simulink model "BMSStateMachine"  (R2023b)
settings: Solver=FixedStepDiscrete  StartTime=0.0  StopTime=10000  RelTol=1e-3
model workspace (MAT data in the model file):
  CV_Gain = 0.20000000298
  HighTempLimit = 50
  I_cc = 30
  LowTempLimit = 5
  MaxCellVoltThrsld = 4.19999980927
  OverCellVoltageLimit = 4.19999980927
  SnsrFltThld = 0.252
  UnderCellVoltageLimit = 2.5
  contactorTime = 200
  currentFactor = 10
  noCurrent = 0
  timeoutContactor = 1
  timeoutCurrent = 1
  vRatio = 0.949999988079
  voltThreshold = 4.09999990463
settings Model: DataDictionary=VirtualVehicleTemplate.sldd  ModifiedByFormat=The MathWorks, Inc.  ExtModeTrigDuration=5  Creator=The MathWorks, Inc.  LastModifiedBy=The MathWorks, Inc.
settings SolverCC: AlgebraicLoopSolver=TrustRegion  PositivePriorityOrder=on  AutoInsertRateTranBlk=on  MaxZcPerStep=1
settings DataIOCC: ExternalInput=Battery  SaveOutput=off  SaveTime=off  SignalLoggingName=logsOut
settings OptimizationCC: BlockReduction=off  DefaultParameterBehavior=Inlined  UseFloatMulNetSlope=on  DefaultUnderspecifiedDataType=single  OptimizeBlockIOStorage=off  EnhancedBackFolding=on  PassReuseOutputArgsThreshold=0  ZeroExternalMemoryAtStartup=off  ZeroInternalMemoryAtStartup=off  EfficientFloat2IntCast=on  MaxStackSize=64  OptimizeBlockOrder=speed  DifferentSizesBufferReuse=on
settings DebuggingCC: SignalInfNanChecking=error  SaveWithParameterizedLinksMsg=none  CheckExecutionContextPreStartOutputMsg=on  IntegerOverflowMsg=error  ParameterPrecisionLossMsg=none  ParameterTunabilityLossMsg=error  UnconnectedInputMsg=warning  UnconnectedOutputMsg=warning  UnconnectedLineMsg=warning  AssertControl=DisableAll  PregeneratedLibrarySubsystemCodeDiagnostic=none  SubsystemReferenceDiagnosticForUnitTest=warning  SFUnexpectedBacktrackingDiag=warning  SFNoUnconditionalDefaultTransitionDiag=warning  SFExecutionAtInitializationDiag=none  ArithmeticOperatorsInVariantConditions=warning
settings HardwareCC: ProdBitPerLong=64  ProdLongLongMode=on  ProdHWDeviceType=Intel->x86-64 (Linux 64)
settings ModelReferenceCC: EnableRefExpFcnMdlSchedulingChecks=on  ModelReferenceNumInstancesAllowed=Single  PropagateSignalLabelsOutOfModel=off
settings SFSimCC: SimUseLocalCustomCode=off  MATLABDynamicMemAlloc=off  CustomCodeUndefinedFunction=UseInterfaceOnly
settings RTWCC: GenerateReport=on  RTWUseLocalCustomCode=off  Toolchain=Simulink Real-Time Toolchain  BuildConfiguration=Faster Runs  TargetLang=C++  DLArmComputeVersion=19.05
settings CodeAppCC: ForceParamTrailComments=on  MaxIdLength=51  OperatorAnnotations=on  MangleLength=4
settings GRTTargetCC: TargetLangStandard=C++03 (ISO)  CodeInterfacePackaging=C++ class
settings ConfigComp: CovMetricSettings=dcw  CovSaveCumulativeToWorkspaceVar=on  CovSaveSingleToWorkspaceVar=on  CovExternalEMLEnable=off  CovSFcnEnable=off  DVMode=DesignErrorDetection  DVMaxProcessTime=7000  DVTestSuiteOptimization=Auto  DVDetectDeadLogic=on  DVDetectIntegerOverflow=off

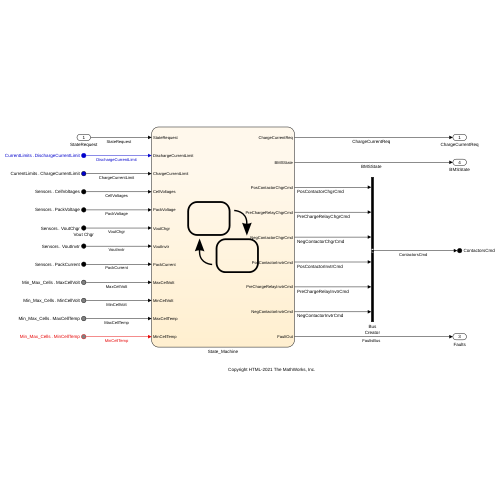
[thumbnail: Simulink's stored preview of the top-level diagram]
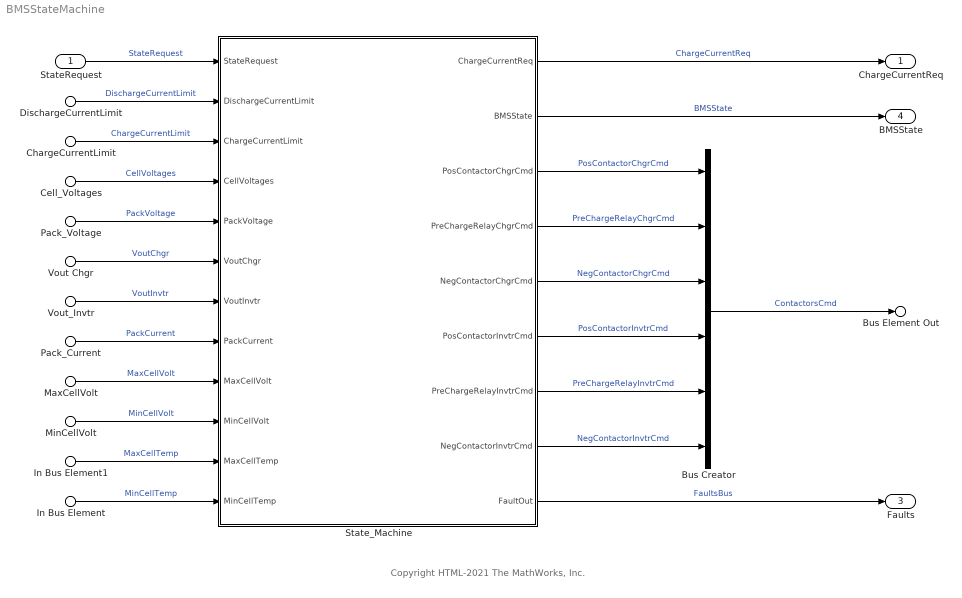
== system BMSStateMachine ==
  note: Copyright HTML-2021 The MathWorks, Inc.
  StateRequest : Inport  OutDataTypeStr=single  PortDimensions=1  SampleTime=[0.10000000000000001,0]
  Cell_Voltages : Inport  Port=2  PortName=Sensors  Element=CellVoltages
  Pack_Voltage : Inport  Port=2  PortName=Sensors  Element=PackVoltage
  Pack_Current : Inport  Port=2  PortName=Sensors  Element=PackCurrent
  Vout Chgr : Inport  Port=2  PortName=Sensors  Element=VoutChgr
  Vout_Invtr : Inport  Port=2  PortName=Sensors  Element=VoutInvtr
  DischargeCurrentLimit : Inport  Port=3  PortName=CurrentLimits  Element=DischargeCurrentLimit
  ChargeCurrentLimit : Inport  Port=3  PortName=CurrentLimits  Element=ChargeCurrentLimit
  MinCellVolt : Inport  Port=4  PortName=Min_Max_Cells  Element=MinCellVolt
  MaxCellVolt : Inport  Port=4  PortName=Min_Max_Cells  Element=MaxCellVolt
  In Bus Element : Inport  Port=4  PortName=Min_Max_Cells  Element=MinCellTemp
  In Bus Element1 : Inport  Port=4  PortName=Min_Max_Cells  Element=MaxCellTemp
  Bus Creator : BusCreator  Inputs=6
  State_Machine : Stateflow chart  TreatAsAtomicUnit=on  VariantControl=(default)
  ChargeCurrentReq : Outport  OutMin=-100  OutMax=100  OutDataTypeStr=single  PortDimensions=1  SampleTime=[0.10000000000000001,0]  VectorParamsAs1DForOutWhenUnconnected=off
  Bus Element Out : Outport  Port=2  PortName=ContactorsCmd
  Faults : Outport  Port=3  OutDataTypeStr=boolean
  BMSState : Outport  Port=4  OutDataTypeStr=single  PortDimensions=1  SampleTime=[0.10000000000000001,0]  VectorParamsAs1DForOutWhenUnconnected=off
  wires:
  Pack_Voltage/1 -> State_Machine/5(PackVoltage)  "PackVoltage"
  Vout_Invtr/1 -> State_Machine/7(VoutInvtr)  "VoutInvtr"
  In Bus Element/1 -> State_Machine/12(MinCellTemp)  "MinCellTemp"
  In Bus Element1/1 -> State_Machine/11(MaxCellTemp)  "MaxCellTemp"
  State_Machine/8(NegContactorInvtrCmd) -> Bus Creator/6  "NegContactorInvtrCmd"
  DischargeCurrentLimit/1 -> State_Machine/2(DischargeCurrentLimit)  "DischargeCurrentLimit"
  State_Machine/2(BMSState) -> BMSState/1  "BMSState"
  State_Machine/6(PosContactorInvtrCmd) -> Bus Creator/4  "PosContactorInvtrCmd"
  Vout Chgr/1 -> State_Machine/6(VoutChgr)  "VoutChgr"
  Pack_Current/1 -> State_Machine/8(PackCurrent)  "PackCurrent"
  MaxCellVolt/1 -> State_Machine/9(MaxCellVolt)  "MaxCellVolt"
  ChargeCurrentLimit/1 -> State_Machine/3(ChargeCurrentLimit)  "ChargeCurrentLimit"
  Bus Creator/1 -> Bus Element Out/1  "ContactorsCmd"
  State_Machine/9(FaultOut) -> Faults/1  "FaultsBus"
  State_Machine/7(PreChargeRelayInvtrCmd) -> Bus Creator/5  "PreChargeRelayInvtrCmd"
  MinCellVolt/1 -> State_Machine/10(MinCellVolt)  "MinCellVolt"
  State_Machine/1(ChargeCurrentReq) -> ChargeCurrentReq/1  "ChargeCurrentReq"
  State_Machine/4(PreChargeRelayChgrCmd) -> Bus Creator/2  "PreChargeRelayChgrCmd"
  State_Machine/3(PosContactorChgrCmd) -> Bus Creator/1  "PosContactorChgrCmd"
  Cell_Voltages/1 -> State_Machine/4(CellVoltages)  "CellVoltages"
  StateRequest/1 -> State_Machine/1(StateRequest)  "StateRequest"
  State_Machine/5(NegContactorChgrCmd) -> Bus Creator/3  "NegContactorChgrCmd"

== stateflow chart BMSStateMachine/State_Machine ==
  state Fault Monitoring [group]
    state MonitorCurrLim [parallel]
      settings: executionOrder=1
      state Wait
      state NoCurrLimFault
      state OverCurrentFault
        en:
        FaultPresent = true;
        FaultOut = true;
      (default) -> NoCurrLimFault : {FaultPresent = false;
          | FaultOut = false;}
      NoCurrLimFault -> Wait : [(PackCurrent < DischargeCurrentLimit) || ...
          | (PackCurrent > ChargeCurrentLimit)]
      Wait -> NoCurrLimFault [order 2] : [(PackCurrent >= DischargeCurrentLimit) && ...
          | (PackCurrent <= ChargeCurrentLimit)]
      Wait -> OverCurrentFault [order 1] : [after(timeoutCurrent,sec)]
    state MonitorCellVoltage [parallel]
      settings: executionOrder=2
      state OverVoltageFault
        en:
        FaultPresent = true;
        FaultOut = true;
      state NoCellVoltFault
        en,du:
        Delta = abs(PackVoltage - sum(CellVoltages));
      state SensorFaut
        en:
        FaultPresent = true;
        FaultOut = true;
      state UnderVoltageFault
        en:
        FaultPresent = true;
        FaultOut = true;
      (default) -> NoCellVoltFault : {FaultPresent = false;
          | FaultOut = false;
          | }
      NoCellVoltFault -> OverVoltageFault [order 1] : [MaxCellVolt >= ...
          | OverCellVoltageLimit]
      NoCellVoltFault -> SensorFaut [order 2] : [Delta >=...
          |  single(SnsrFltThld)]
      NoCellVoltFault -> UnderVoltageFault [order 3] : [MinCellVolt <=...
          |  UnderCellVoltageLimit]
    state MonitorCellTemp [parallel]
      settings: executionOrder=3
      state HighTemperatureFault
        en:
        FaultPresent = true;
        FaultOut = true;
      state NoCellTempFault
      state LowTemperatureFault
        en:
        FaultPresent = true;
        FaultOut = true;
      (default) -> NoCellTempFault : {FaultPresent = false;
          | FaultOut = false;}
      NoCellTempFault -> HighTemperatureFault [order 1] : [MaxCellTemp >= HighTempLimit]
      NoCellTempFault -> LowTemperatureFault [order 2] : [MinCellTemp <= LowTempLimit]
  state MainStateMachine [parallel]
    settings: executionOrder=1
    state Charging
      en:
      BMSState = 1;
      state Init_Mode
        en:
        ChargeModeReq = 0;
        ChargeCurrentReq = noCurrent;
      state CC_Mode
        en:
        ChargeModeReq = 1;
        du:
        ChargeCurrentReq = min(I_cc,ChargeCurrentLimit);
      state CV_Mode
        en:
        ChargeModeReq = 2;
        du:
        ChargeCurrentReq = ChargeCurrentReq - CV_Gain*(MaxCellVolt - MaxCellVoltThrsld);
        ChargeCurrentReq = min(ChargeCurrentReq, ChargeCurrentLimit);
      (default) -> Init_Mode
      CV_Mode -> Init_Mode : [StateRequest ~= 1 || ...
          | ChargeCurrentReq <= (I_cc/currentFactor)]
      CC_Mode -> Init_Mode [order 1] : [StateRequest ~= 1]
      Init_Mode -> CC_Mode : [StateRequest == 1 && ...
          | MaxCellVolt < voltThreshold]
      CC_Mode -> CV_Mode [order 2] : [MaxCellVolt>=...
          | MaxCellVoltThrsld]
    state Standby
      en:
      BMSState = ...
      0;
    state Driving
      en:
      BMSState = ...
      2;
    state Fault
      en,du:
      BMSState = 3;
    (default) -> Standby
    Standby -> (junction 577) [order 1] : [FaultPresent]
    Standby -> Charging [order 2] : [StateRequest ==1 ...
        | && ChrgCntctState == Contact.Close]
    (junction 577) -> (junction 580)
    Charging -> Standby [order 3] : [StateRequest ~=1 ...
        |  && ChrgCntctState == Contact.Init]
    Standby -> Driving [order 3] : [StateRequest == 2 && ...
        | InvtrCntctState == Contact.Close]
    Driving -> Standby [order 3] : [StateRequest ~= 2 && ...
        | InvtrCntctState == Contact.Init]
    Driving -> Charging [order 2] : [StateRequest == 1 && ...
        | ChrgCntctState == Contact.Close]
    Charging -> Driving [order 2] : [StateRequest == 2 && ...
        | InvtrCntctState == Contact.Close]
    Driving -> Fault [order 1] : [FaultPresent]
    Charging -> Fault [order 1] : [FaultPresent]{ChargeCurrentReq = single(0);}
    (junction 580) -> Fault
  state ChargerContactorState [parallel]
    settings: executionOrder=2
    state OpenChgrContactors
      state ClosePreChrgRly
        PreChargeRelayChgrCmd = true;
      state OpenPosCntct
        PosContactorChgrCmd = false;
      state OpenPreChrgRly
        PreChargeRelayChgrCmd = false;
      state OpenNegCntct
        NegContactorChgrCmd = false;
        ChrgCntctState = Contact.Open;
        PreChrgFault = false;
        FaultOut = false;
      (default) -> ChargerContactorState.OpenChgrContactors.ClosePreChrgRly : {ChrgCntctState = Contact.Init;}
      ChargerContactorState.OpenChgrContactors.ClosePreChrgRly -> ChargerContactorState.OpenChgrContactors.OpenPosCntct : after(contactorTime,msec) % Check for low current
      ChargerContactorState.OpenChgrContactors.OpenPosCntct -> ChargerContactorState.OpenChgrContactors.OpenPreChrgRly : after(contactorTime,msec)
      ChargerContactorState.OpenChgrContactors.OpenPreChrgRly -> ChargerContactorState.OpenChgrContactors.OpenNegCntct : after(contactorTime,msec)
    state CloseChgrContactors
      state CloseNegCntct
        NegContactorChgrCmd = true;
      state ClosePreChrgRly
        PreChargeRelayChgrCmd = true;
      state ClosePosCntct
        PosContactorChgrCmd = true;
      state OpenPreChrgRly
        PreChargeRelayChgrCmd = false;
        ChrgCntctState = Contact.Close;
      state PreChrgFlt
        PreChrgFault = true;
        FaultOut = true;
      (default) -> ChargerContactorState.CloseChgrContactors.CloseNegCntct : {ChrgCntctState = Contact.Init;}
      ChargerContactorState.CloseChgrContactors.CloseNegCntct -> ChargerContactorState.CloseChgrContactors.ClosePreChrgRly : after(contactorTime,msec)
      ChargerContactorState.CloseChgrContactors.ClosePreChrgRly -> (junction 564) [order 2]
      (junction 564) -> (junction 566) : after(timeoutContactor,sec)
          | % Check timeout
      ChargerContactorState.CloseChgrContactors.ClosePreChrgRly -> ChargerContactorState.CloseChgrContactors.ClosePosCntct [order 1] : [VoutChgr/PackVoltage >=vRatio]
      ChargerContactorState.CloseChgrContactors.ClosePosCntct -> ChargerContactorState.CloseChgrContactors.OpenPreChrgRly : after(contactorTime,msec)
      (junction 566) -> ChargerContactorState.CloseChgrContactors.PreChrgFlt
    (default) -> OpenChgrContactors : {ChrgCntctState = Contact.Init;
        | PreChrgFault = false;
        | FaultOut = false;}
    CloseChgrContactors -> OpenChgrContactors : [StateRequest ~= 1 || ...
        | FaultPresent]
    OpenChgrContactors -> CloseChgrContactors : [StateRequest == 1 && ...
        | InvtrCntctState == Contact.Open && ...
        | ~FaultPresent]
  state InverterContactorState [parallel]
    settings: executionOrder=3
    state CloseInvtrContactors
      state CloseNegCntct
        NegContactorInvtrCmd = true;
      state ClosePreChrgRly
        PreChargeRelayInvtrCmd = true;
      state ClosePosCntct
        PosContactorInvtrCmd = true;
      state OpenPreChrgRly
        PreChargeRelayInvtrCmd = false;
        InvtrCntctState = Contact.Close;
      state PreChrgFlt
        PreChrgFault = true;
        FaultOut = true;
      (default) -> InverterContactorState.CloseInvtrContactors.CloseNegCntct : {InvtrCntctState = Contact.Init;}
      InverterContactorState.CloseInvtrContactors.CloseNegCntct -> InverterContactorState.CloseInvtrContactors.ClosePreChrgRly : after(contactorTime,msec)
      InverterContactorState.CloseInvtrContactors.ClosePreChrgRly -> (junction 569) [order 2]
      (junction 569) -> (junction 570) : after(timeoutContactor,sec)
          | % Check timeout
      InverterContactorState.CloseInvtrContactors.ClosePreChrgRly -> InverterContactorState.CloseInvtrContactors.ClosePosCntct [order 1] : [VoutInvtr/PackVoltage >=vRatio]
      InverterContactorState.CloseInvtrContactors.ClosePosCntct -> InverterContactorState.CloseInvtrContactors.OpenPreChrgRly : after(contactorTime,msec)
      (junction 570) -> InverterContactorState.CloseInvtrContactors.PreChrgFlt
    state OpenInvtrContactors
      state ClosePreChrgRly
        PreChargeRelayInvtrCmd = true;
      state OpenPosCntct
        PosContactorInvtrCmd = false;
      state OpenPreChrgRly
        PreChargeRelayInvtrCmd = false;
      state OpenNegCntct
        NegContactorInvtrCmd = false;
        InvtrCntctState = Contact.Open;
        PreChrgFault = false;
        FaultOut = false;
      (default) -> InverterContactorState.OpenInvtrContactors.ClosePreChrgRly : {InvtrCntctState = Contact.Init;}
      InverterContactorState.OpenInvtrContactors.ClosePreChrgRly -> InverterContactorState.OpenInvtrContactors.OpenPosCntct : after(contactorTime,msec) % Check for low current
      InverterContactorState.OpenInvtrContactors.OpenPosCntct -> InverterContactorState.OpenInvtrContactors.OpenPreChrgRly : after(contactorTime,msec)
      InverterContactorState.OpenInvtrContactors.OpenPreChrgRly -> InverterContactorState.OpenInvtrContactors.OpenNegCntct : after(contactorTime,msec)
    (default) -> OpenInvtrContactors : {InvtrCntctState =Contact.Init;
        | PreChrgFault = false;
        | FaultOut = false;}
    CloseInvtrContactors -> OpenInvtrContactors : [StateRequest ~= 2 || ...
        | FaultPresent]
    OpenInvtrContactors -> CloseInvtrContactors : [StateRequest == 2 && ...
        | ChrgCntctState == Contact.Open && ...
        | ~FaultPresent]
  data: StateRequest input; DischargeCurrentLimit input single; ChargeCurrentLimit input single; CellVoltages input single; PackVoltage input single; VoutChgr input single; VoutInvtr input single; PackCurrent input single; ChargeCurrentReq output; I_cc parameter; MaxCellVolt input single; BMSState output single =single(0); PosContactorChgrCmd output boolean; PreChargeRelayChgrCmd output; NegContactorChgrCmd output; PosContactorInvtrCmd output; PreChargeRelayInvtrCmd output; NegContactorInvtrCmd output; ChrgCntctState local Enum: Contact; InvtrCntctState local Enum: Contact; PreChrgFault local; MaxCellVoltThrsld parameter; FaultPresent local; MinCellVolt input single; OverCellVoltageLimit parameter; UnderCellVoltageLimit parameter; Delta local; HighTempLimit parameter; LowTempLimit parameter; SnsrFltThld parameter; CV_Gain parameter; ChargeModeReq local =0; MonitorCurrLimMode local Enum: MonitorCurrLimModeType; MonitorCellVoltageMode local Enum: MonitorCellVoltageModeType; MonitorCellTempMode local Enum: MonitorCellTempModeType; FaultOut output boolean; contactorTime parameter uint16; timeoutContactor parameter uint8; timeoutCurrent parameter uint8; vRatio parameter single; voltThreshold parameter single; currentFactor parameter single; noCurrent parameter single; MaxCellTemp input; MinCellTemp input
